simulink model "GS_model"  (R2018b)
settings: Solver=ode5  StartTime=0.0  StopTime=SimuStopTime  FixedStep=T_Simu  RelTol=1e-3
InitFcn:
  | Initial
undefined symbols (not defined in the file or in its folder): Aba10, Aba20, aeroCIP2006_S, aeroCIP2006_X, aeroCIP2006_Y, Agl0, Ass_kS, Ass_n1, Ass_n2, Ass_n3, Ass_n4, Ass_Noise, Ass_R, Ass_Resolution, Ass_TmOrder, AssA_Fix_Abs, AssB_Fix_Abs, AssC_Fix_Abs, AssD_Fix_Abs, AssE_Fix_Aps, AssF_Fix_Aps, C, c_max, c_min, Cd, CenterOfFigNX, CenterOfFigNY, CenterOfFigNZ, CenterOfFigP1, CenterOfFigP2, CenterOfFigPX, CenterOfFigPY, CenterOfFigPZ, Cmu, Crou, DEG2RAD, DiscIntNeverNeededParam, Eg_Dir, Eg_F, Eg_PrepareTime, Eg_r_L_L, Fw_Abf, Fw_Hmax, Fw_J, Fw_Spd0, Fw_Tmax, git_hash_BaseLine, git_hash_Project, Gnss_Noise_Pos, Gnss_Noise_Vel, Gnss_PropgationTime, GyroA_Fix_Abg, GyroA_Noise, GyroB_Fix_Abg, GyroB_Noise, GyroC_Fix_Abg, GyroC_Noise, GyroD_Fix_Abg, GyroD_Noise, h ... (+94)
libraries: simulink x308, sharedutil x46, aerolibutil x37, sharedtransform x31, vrlib x14, aerolibgravity2 x2
(part 4 of 20)

== system GS_model/Subsystem2/EquipmentCmd/Fw1/Subsystem7/Subsystem3 ==
  note: 1 -- FW_Spd_422
      | 2 -- FW_Spd_UDP
      | 3 -- FW_Spd_FC
      |
      | 4 -- FW_T_422
      | 5 -- FW_T_UDP
      | 6 -- FW_T_FC
      |
      | 7 -- FW_Mode_422
      | 8 -- FW_Mode_UDP
      | 9 -- FW_Mode_FC
      |
      | 10--FW_DataSource
  note: FW_DataSource
      | AA-真采集（默认）  1-422(DB9);
      |                                  0-反测（默认
      | 55 -伪采集                UDP
  FWNum : Inport
  FW_Cmd : Inport  Port=2
  TC_Fw : Inport  Port=3
  Compare To Constant : simulink/Logic and Bit Operations/Compare To Constant  relop===  const=0  OutDataTypeStr=boolean
  Demux : Demux  Outputs=[9;1]
  Demux2 : Demux  Outputs=[1;2]
  FWDataSourceChoice : Subsystem
      mask Display: disp('FWDataSourceChoice')
  Logical Operator : Logic  Operator=OR  AllPortsSameDT=off  OutDataTypeStr=boolean
  Mux : Mux  Inputs=3
  Mux1 : Mux  Inputs=2
  Relational Operator1 : RelationalOperator  Operator===  OutDataTypeStr=boolean  RndMeth=Simplest
  Selector : Selector  InputPortWidth=3  IndexOptions=Index vector (dialog)  Indices=[2 3 1]  OutputSizes=1
  Selector2 : Selector  InputPortWidth=23  IndexOptions=Index vector (dialog)  Indices=[1 2]  OutputSizes=1
  Triggered Subsystem1 : Subsystem  TreatAsAtomicUnit=on
      mask Display: disp('FWChoice')
  Cmd_Mode/Spd/T : Outport
  wires:
  Mux/1 -> Cmd_Mode/Spd/T/1
  FWDataSourceChoice/1(Cmd_Mode) -> Mux/1
  Demux/1 -> FWDataSourceChoice/2(FW_Cmd)
  Demux/2 -> Mux1/1
  FW_Cmd/1 -> Demux/1
  TC_Fw/1 -> Selector2/1
  Selector2/1 -> Mux1/2
  FWDataSourceChoice/3(Cmd_T) -> Mux/3
  FWDataSourceChoice/2(Cmd_Spd) -> Mux/2
  Compare To Constant/1 -> Logical Operator/2
  Triggered Subsystem1/1(Out1) -> FWDataSourceChoice/1(FW_Data_Source)
  Mux1/1 -> Selector/1
  Demux2/2 -> Triggered Subsystem1/1(In1)
  Selector/1 -> Demux2/1
  Relational Operator1/1 -> Logical Operator/1
  Logical Operator/1 -> Triggered Subsystem1/Enable
  Demux2/1 -> Compare To Constant/1, Relational Operator1/2
  FWNum/1 -> Relational Operator1/1

== system GS_model/Subsystem2/EquipmentCmd/Fw1/Subsystem7/Subsystem4 ==
  note: FW_DataSource
      | AA-真采集（默认）  1-422(DB9);
      |                                  0-反测（默认
      | 55 -伪采集                UDP
  note: 1 -- FW_Spd_422
      | 2 -- FW_Spd_UDP
      | 3 -- FW_Spd_FC
      |
      | 4 -- FW_T_422
      | 5 -- FW_T_UDP
      | 6 -- FW_T_FC
      |
      | 7 -- FW_Mode_422
      | 8 -- FW_Mode_UDP
      | 9 -- FW_Mode_FC
      |
      | 10--FW_DataSource
  FWNum : Inport
  FW_Cmd : Inport  Port=2
  TC_Fw : Inport  Port=3
  Compare To Constant : simulink/Logic and Bit Operations/Compare To Constant  relop===  const=0  OutDataTypeStr=boolean
  Demux : Demux  Outputs=[9;1]
  Demux2 : Demux  Outputs=[1;2]
  FWDataSourceChoice : Subsystem
      mask Display: disp('FWDataSourceChoice')
  Logical Operator : Logic  Operator=OR  AllPortsSameDT=off  OutDataTypeStr=boolean
  Mux : Mux  Inputs=3
  Mux1 : Mux  Inputs=2
  Relational Operator1 : RelationalOperator  Operator===  OutDataTypeStr=boolean  RndMeth=Simplest
  Selector : Selector  InputPortWidth=3  IndexOptions=Index vector (dialog)  Indices=[2 3 1]  OutputSizes=1
  Selector2 : Selector  InputPortWidth=23  IndexOptions=Index vector (dialog)  Indices=[1 2]  OutputSizes=1
  Triggered Subsystem1 : Subsystem  TreatAsAtomicUnit=on
      mask Display: disp('FWChoice')
  Cmd_Mode/Spd/T : Outport
  wires:
  FWNum/1 -> Relational Operator1/1
  Demux2/1 -> Relational Operator1/2, Compare To Constant/1
  Logical Operator/1 -> Triggered Subsystem1/Enable
  Relational Operator1/1 -> Logical Operator/1
  Selector/1 -> Demux2/1
  Demux2/2 -> Triggered Subsystem1/1(In1)
  Mux1/1 -> Selector/1
  Triggered Subsystem1/1(Out1) -> FWDataSourceChoice/1(FW_Data_Source)
  Compare To Constant/1 -> Logical Operator/2
  FWDataSourceChoice/2(Cmd_Spd) -> Mux/2
  FWDataSourceChoice/3(Cmd_T) -> Mux/3
  Selector2/1 -> Mux1/2
  TC_Fw/1 -> Selector2/1
  FW_Cmd/1 -> Demux/1
  Demux/2 -> Mux1/1
  Demux/1 -> FWDataSourceChoice/2(FW_Cmd)
  FWDataSourceChoice/1(Cmd_Mode) -> Mux/1
  Mux/1 -> Cmd_Mode/Spd/T/1

== system GS_model/Subsystem2/EquipmentCmd/Fw1/Subsystem7/Subsystem5 ==
  note: 1 -- FW_Spd_422
      | 2 -- FW_Spd_UDP
      | 3 -- FW_Spd_FC
      |
      | 4 -- FW_T_422
      | 5 -- FW_T_UDP
      | 6 -- FW_T_FC
      |
      | 7 -- FW_Mode_422
      | 8 -- FW_Mode_UDP
      | 9 -- FW_Mode_FC
      |
      | 10--FW_DataSource
  note: FW_DataSource
      | AA-真采集（默认）  1-422(DB9);
      |                                  0-反测（默认
      | 55 -伪采集                UDP
  FWNum : Inport
  FW_Cmd : Inport  Port=2
  TC_Fw : Inport  Port=3
  Compare To Constant : simulink/Logic and Bit Operations/Compare To Constant  relop===  const=0  OutDataTypeStr=boolean
  Demux : Demux  Outputs=[9;1]
  Demux2 : Demux  Outputs=[1;2]
  FWDataSourceChoice : Subsystem
      mask Display: disp('FWDataSourceChoice')
  Logical Operator : Logic  Operator=OR  AllPortsSameDT=off  OutDataTypeStr=boolean
  Mux : Mux  Inputs=3
  Mux1 : Mux  Inputs=2
  Relational Operator1 : RelationalOperator  Operator===  OutDataTypeStr=boolean  RndMeth=Simplest
  Selector : Selector  InputPortWidth=3  IndexOptions=Index vector (dialog)  Indices=[2 3 1]  OutputSizes=1
  Selector2 : Selector  InputPortWidth=23  IndexOptions=Index vector (dialog)  Indices=[1 2]  OutputSizes=1
  Triggered Subsystem1 : Subsystem  TreatAsAtomicUnit=on
      mask Display: disp('FWChoice')
  Cmd_Mode/Spd/T : Outport
  wires:
  Mux/1 -> Cmd_Mode/Spd/T/1
  FWDataSourceChoice/1(Cmd_Mode) -> Mux/1
  Demux/1 -> FWDataSourceChoice/2(FW_Cmd)
  Demux/2 -> Mux1/1
  FW_Cmd/1 -> Demux/1
  TC_Fw/1 -> Selector2/1
  Selector2/1 -> Mux1/2
  FWDataSourceChoice/3(Cmd_T) -> Mux/3
  FWDataSourceChoice/2(Cmd_Spd) -> Mux/2
  Compare To Constant/1 -> Logical Operator/2
  Triggered Subsystem1/1(Out1) -> FWDataSourceChoice/1(FW_Data_Source)
  Mux1/1 -> Selector/1
  Demux2/2 -> Triggered Subsystem1/1(In1)
  Selector/1 -> Demux2/1
  Relational Operator1/1 -> Logical Operator/1
  Logical Operator/1 -> Triggered Subsystem1/Enable
  Demux2/1 -> Compare To Constant/1, Relational Operator1/2
  FWNum/1 -> Relational Operator1/1

== system GS_model/Subsystem2/EquipmentCmd/Fw1/Subsystem7/Subsystem6 ==
  note: FW_DataSource
      | AA-真采集（默认）  1-422(DB9);
      |                                  0-反测（默认
      | 55 -伪采集                UDP
  note: 1 -- FW_Spd_422
      | 2 -- FW_Spd_UDP
      | 3 -- FW_Spd_FC
      |
      | 4 -- FW_T_422
      | 5 -- FW_T_UDP
      | 6 -- FW_T_FC
      |
      | 7 -- FW_Mode_422
      | 8 -- FW_Mode_UDP
      | 9 -- FW_Mode_FC
      |
      | 10--FW_DataSource
  FWNum : Inport
  FW_Cmd : Inport  Port=2
  TC_Fw : Inport  Port=3
  Compare To Constant : simulink/Logic and Bit Operations/Compare To Constant  relop===  const=0  OutDataTypeStr=boolean
  Demux : Demux  Outputs=[9;1]
  Demux2 : Demux  Outputs=[1;2]
  FWDataSourceChoice : Subsystem
      mask Display: disp('FWDataSourceChoice')
  Logical Operator : Logic  Operator=OR  AllPortsSameDT=off  OutDataTypeStr=boolean
  Mux : Mux  Inputs=3
  Mux1 : Mux  Inputs=2
  Relational Operator1 : RelationalOperator  Operator===  OutDataTypeStr=boolean  RndMeth=Simplest
  Selector : Selector  InputPortWidth=3  IndexOptions=Index vector (dialog)  Indices=[2 3 1]  OutputSizes=1
  Selector2 : Selector  InputPortWidth=23  IndexOptions=Index vector (dialog)  Indices=[1 2]  OutputSizes=1
  Triggered Subsystem1 : Subsystem  TreatAsAtomicUnit=on
      mask Display: disp('FWChoice')
  Cmd_Mode/Spd/T : Outport
  wires:
  FWNum/1 -> Relational Operator1/1
  Demux2/1 -> Relational Operator1/2, Compare To Constant/1
  Logical Operator/1 -> Triggered Subsystem1/Enable
  Relational Operator1/1 -> Logical Operator/1
  Selector/1 -> Demux2/1
  Demux2/2 -> Triggered Subsystem1/1(In1)
  Mux1/1 -> Selector/1
  Triggered Subsystem1/1(Out1) -> FWDataSourceChoice/1(FW_Data_Source)
  Compare To Constant/1 -> Logical Operator/2
  FWDataSourceChoice/2(Cmd_Spd) -> Mux/2
  FWDataSourceChoice/3(Cmd_T) -> Mux/3
  Selector2/1 -> Mux1/2
  TC_Fw/1 -> Selector2/1
  FW_Cmd/1 -> Demux/1
  Demux/2 -> Mux1/1
  Demux/1 -> FWDataSourceChoice/2(FW_Cmd)
  FWDataSourceChoice/1(Cmd_Mode) -> Mux/1
  Mux/1 -> Cmd_Mode/Spd/T/1

== system GS_model/Subsystem2/Subsystem/Actuator/Engine/Subsystem ==
  note: F_Choice/Switch/Value
  note: Dir_Choice/Switch/X/Y/Z
  note: FirePause_Choice/Switch/Value
  Tc_F_Engine : Inport
  Cmd_Engine : Inport  Port=2
  Cent : Inport  Port=3
  Eg_F : Inport  Port=4
  Eg_PrepareTime : Inport  Port=5
  Eg_r_L_L : Inport  Port=6
  Eg_Dir : Inport  Port=7
  EgNum : Inport  Port=8
  Demux1 : Demux  Outputs=[5;3;3]
  Engine : Subsystem
      mask Display: disp('EngineModel')
  Fcn : Fcn  Expr=3*u(1)-2
  Fcn1 : Fcn  Expr=3*u(1)-2
  Fcn2 : Fcn  Expr=2*u(1)-1
  Fcn3 : Fcn  Expr=2*u(1)
  Selector1 : Selector  InputPortWidth=size(Eg_F,1)  IndexOptions=Starting index (port)  Indices=[1 3]  OutputSizes=1
  Selector14 : Selector  InputPortWidth=size(Eg_F,1)*2  IndexOptions=Starting index (port)  Indices=[1 3]  OutputSizes=1
  Selector2 : Selector  InputPortWidth=size(Eg_F,1)  IndexOptions=Starting index (port)  Indices=[1 3]  OutputSizes=1
  Selector3 : Selector  InputPortWidth=size(Eg_F,1)*3  IndexOptions=Starting index (port)  Indices=[1 3]  OutputSizes=3
  Selector4 : Selector  InputPortWidth=size(Eg_F,1)*3  IndexOptions=Starting index (port)  Indices=[1 3]  OutputSizes=3
  Selector5 : Selector  InputPortWidth=size(Eg_F,1)*2  IndexOptions=Starting index (port)  Indices=[1 3]  OutputSizes=1
  Subsystem : Subsystem
  Subsystem1 : Subsystem
  Subsystem2 : Subsystem
  T : Outport
  F : Outport  Port=2
  wires:
  Engine/2(F_EP) -> F/1
  Engine/1(T_Engine) -> T/1
  EgNum/1 -> Fcn2/1, Fcn3/1, Selector1/2, Subsystem2/2(Num), Subsystem1/3(Num), Subsystem/3(Num), Selector2/2, Fcn1/1, Fcn/1
  Cent/1 -> Engine/5(Cent)
  Eg_PrepareTime/1 -> Selector1/1
  Tc_F_Engine/1 -> Demux1/1
  Demux1/2 -> Subsystem1/2(Eg_F_Set)
  Eg_r_L_L/1 -> Selector3/1
  Fcn/1 -> Selector3/2
  Selector1/1 -> Engine/3(Eg_PrepareTime)
  Selector3/1 -> Engine/4(Eg_r_L_L)
  Fcn1/1 -> Selector4/2
  Eg_Dir/1 -> Selector4/1
  Selector4/1 -> Subsystem/1(Eg_Dir0)
  Demux1/1 -> Subsystem/2(Eg_Dir_Set)
  Selector2/1 -> Subsystem1/1(Eg_F0)
  Eg_F/1 -> Selector2/1
  Subsystem/1(Eg_Dir) -> Engine/6(Eg_Dir)
  Subsystem1/1(Eg_F) -> Engine/7(Eg_F)
  Fcn2/1 -> Selector5/2
  Fcn3/1 -> Selector14/2
  Cmd_Engine/1 -> Selector14/1, Selector5/1
  Selector5/1 -> Engine/1(FireSwitch)
  Selector14/1 -> Engine/2(FireTime)
  Demux1/3 -> Subsystem2/1(Eg_F_Set)
  Subsystem2/1(Eg_FirePause) -> Engine/8(Eg_Fire_Pause)

== system GS_model/Subsystem2/Subsystem/Actuator/Engine/Subsystem1 ==
  note: FirePause_Choice/Switch/Value
  note: Dir_Choice/Switch/X/Y/Z
  note: F_Choice/Switch/Value
  Tc_F_Engine : Inport
  Cmd_Engine : Inport  Port=2
  Cent : Inport  Port=3
  Eg_F : Inport  Port=4
  Eg_PrepareTime : Inport  Port=5
  Eg_r_L_L : Inport  Port=6
  Eg_Dir : Inport  Port=7
  EgNum : Inport  Port=8
  Demux1 : Demux  Outputs=[5;3;3]
  Engine : Subsystem
      mask Display: disp('EngineModel')
  Fcn : Fcn  Expr=3*u(1)-2
  Fcn1 : Fcn  Expr=3*u(1)-2
  Fcn2 : Fcn  Expr=2*u(1)-1
  Fcn3 : Fcn  Expr=2*u(1)
  Selector1 : Selector  InputPortWidth=size(Eg_F,1)  IndexOptions=Starting index (port)  Indices=[1 3]  OutputSizes=1
  Selector14 : Selector  InputPortWidth=size(Eg_F,1)*2  IndexOptions=Starting index (port)  Indices=[1 3]  OutputSizes=1
  Selector2 : Selector  InputPortWidth=size(Eg_F,1)  IndexOptions=Starting index (port)  Indices=[1 3]  OutputSizes=1
  Selector3 : Selector  InputPortWidth=size(Eg_F,1)*3  IndexOptions=Starting index (port)  Indices=[1 3]  OutputSizes=3
  Selector4 : Selector  InputPortWidth=size(Eg_F,1)*3  IndexOptions=Starting index (port)  Indices=[1 3]  OutputSizes=3
  Selector5 : Selector  InputPortWidth=size(Eg_F,1)*2  IndexOptions=Starting index (port)  Indices=[1 3]  OutputSizes=1
  Subsystem : Subsystem
  Subsystem1 : Subsystem
  Subsystem2 : Subsystem
  T : Outport
  F : Outport  Port=2
  wires:
  Subsystem2/1(Eg_FirePause) -> Engine/8(Eg_Fire_Pause)
  Demux1/3 -> Subsystem2/1(Eg_F_Set)
  Selector14/1 -> Engine/2(FireTime)
  Selector5/1 -> Engine/1(FireSwitch)
  Cmd_Engine/1 -> Selector5/1, Selector14/1
  Fcn3/1 -> Selector14/2
  Fcn2/1 -> Selector5/2
  Subsystem1/1(Eg_F) -> Engine/7(Eg_F)
  Subsystem/1(Eg_Dir) -> Engine/6(Eg_Dir)
  Eg_F/1 -> Selector2/1
  Selector2/1 -> Subsystem1/1(Eg_F0)
  Demux1/1 -> Subsystem/2(Eg_Dir_Set)
  Selector4/1 -> Subsystem/1(Eg_Dir0)
  Eg_Dir/1 -> Selector4/1
  Fcn1/1 -> Selector4/2
  Selector3/1 -> Engine/4(Eg_r_L_L)
  Selector1/1 -> Engine/3(Eg_PrepareTime)
  Fcn/1 -> Selector3/2
  Eg_r_L_L/1 -> Selector3/1
  Demux1/2 -> Subsystem1/2(Eg_F_Set)
  Tc_F_Engine/1 -> Demux1/1
  Eg_PrepareTime/1 -> Selector1/1
  Cent/1 -> Engine/5(Cent)
  EgNum/1 -> Fcn/1, Fcn1/1, Selector2/2, Subsystem/3(Num), Subsystem1/3(Num), Subsystem2/2(Num), Selector1/2, Fcn3/1, Fcn2/1
  Engine/1(T_Engine) -> T/1
  Engine/2(F_EP) -> F/1

== system GS_model/Subsystem2/Subsystem/Actuator/FlyWheel/FwAModel1 ==
  note: TC_FW_DelaySet[1*1]
  note: 1 -- TM_FW_Mode
      | 2 -- TM_FW_Spd
      | 3 -- TM_FW_T
      |
      | 4 -- Cmd_FW_Mode
      | 5 -- Cmd_FW_Spd
      | 6 -- Cmd_FW_T
      |
      | 7 -- Dyn_FW_T
      | 8 -- Dyn_FW_Spd
  note: TC_FW_TSet[3*1]
  note: TC_FW_SpdSet[3*1]
  note: TC_FW_ModeSet[3*1]
  note: TC_FWErr_Spd_Op[2*1]
  note: TC_FWErr_T_Op[2*1]
  note: Tc_FW_FricCoffSet[1*1]
  FW_Cmd : Inport
  TC_FW : Inport  Port=2
  FwSpd/T : Inport  Port=3
  FWNum : Inport  Port=4
  Demux : Demux  Outputs=2
  Demux1 : Demux  Outputs=[1;3;3;3;2;2;1]
  FWDataSourceChoice : Subsystem
      mask Display: disp('FWDataSourceChoice')
  FWMath&ErrModel : Subsystem
      mask Display: disp('FWMath&ErrModel')
  Mux : Mux
  Terminator : Terminator
  TM_FW : Outport
  Cmd_Mode/Spd/T : Outport  Port=2
  wires:
  FwSpd/T/1 -> Demux/1
  Demux/2 -> FWMath&ErrModel/8(FwT)
  Demux/1 -> FWMath&ErrModel/7(FwSpd)
  Demux1/7 -> Terminator/1
  FWDataSourceChoice/1(Cmd_Mode/Spd/T) -> Mux/2, Cmd_Mode/Spd/T/1
  Demux1/1 -> FWDataSourceChoice/2(TC_FW_DelaySet)
  FW_Cmd/1 -> FWDataSourceChoice/1(FW_Cmd)
  TC_FW/1 -> Demux1/1
  FWDataSourceChoice/2(Cmd_Mode) -> FWMath&ErrModel/1(Cmd_Mode)
  FWNum/1 -> FWMath&ErrModel/9(FWNum)
  FWMath&ErrModel/1(TM_FW) -> Mux/1
  Demux1/6 -> FWMath&ErrModel/6(TC_FWErr_T_Op)
  Demux1/5 -> FWMath&ErrModel/5(TC_FWErr_Spd_Op)
  Demux1/4 -> FWMath&ErrModel/4(TC_FW_ModeSet)
  Demux1/3 -> FWMath&ErrModel/3(TC_FW_SpdSet)
  Demux1/2 -> FWMath&ErrModel/2(TC_FW_TSet)
  FWMath&ErrModel/2(Dyn_FW_T) -> Mux/3
  Mux/1 -> TM_FW/1
  FWMath&ErrModel/3(Dyn_FW_Spd) -> Mux/4

== system GS_model/Subsystem2/Subsystem/Actuator/FlyWheel/FwAModel2 ==
  note: Tc_FW_FricCoffSet[1*1]
  note: TC_FWErr_T_Op[2*1]
  note: TC_FWErr_Spd_Op[2*1]
  note: TC_FW_ModeSet[3*1]
  note: TC_FW_SpdSet[3*1]
  note: TC_FW_TSet[3*1]
  note: 1 -- TM_FW_Mode
      | 2 -- TM_FW_Spd
      | 3 -- TM_FW_T
      |
      | 4 -- Cmd_FW_Mode
      | 5 -- Cmd_FW_Spd
      | 6 -- Cmd_FW_T
      |
      | 7 -- Dyn_FW_T
      | 8 -- Dyn_FW_Spd
  note: TC_FW_DelaySet[1*1]
  FW_Cmd : Inport
  TC_FW : Inport  Port=2
  FwSpd/T : Inport  Port=3
  FWNum : Inport  Port=4
  Demux : Demux  Outputs=2
  Demux1 : Demux  Outputs=[1;3;3;3;2;2;1]
  FWDataSourceChoice : Subsystem
      mask Display: disp('FWDataSourceChoice')
  FWMath&ErrModel : Subsystem
      mask Display: disp('FWMath&ErrModel')
  Mux : Mux
  Terminator : Terminator
  TM_FW : Outport
  Cmd_Mode/Spd/T : Outport  Port=2
  wires:
  FWMath&ErrModel/3(Dyn_FW_Spd) -> Mux/4
  Mux/1 -> TM_FW/1
  FWMath&ErrModel/2(Dyn_FW_T) -> Mux/3
  Demux1/2 -> FWMath&ErrModel/2(TC_FW_TSet)
  Demux1/3 -> FWMath&ErrModel/3(TC_FW_SpdSet)
  Demux1/4 -> FWMath&ErrModel/4(TC_FW_ModeSet)
  Demux1/5 -> FWMath&ErrModel/5(TC_FWErr_Spd_Op)
  Demux1/6 -> FWMath&ErrModel/6(TC_FWErr_T_Op)
  FWMath&ErrModel/1(TM_FW) -> Mux/1
  FWNum/1 -> FWMath&ErrModel/9(FWNum)
  FWDataSourceChoice/2(Cmd_Mode) -> FWMath&ErrModel/1(Cmd_Mode)
  TC_FW/1 -> Demux1/1
  FW_Cmd/1 -> FWDataSourceChoice/1(FW_Cmd)
  Demux1/1 -> FWDataSourceChoice/2(TC_FW_DelaySet)
  FWDataSourceChoice/1(Cmd_Mode/Spd/T) -> Cmd_Mode/Spd/T/1, Mux/2
  Demux1/7 -> Terminator/1
  Demux/1 -> FWMath&ErrModel/7(FwSpd)
  Demux/2 -> FWMath&ErrModel/8(FwT)
  FwSpd/T/1 -> Demux/1

== system GS_model/Subsystem2/Subsystem/Actuator/FlyWheel/FwAModel3 ==
  note: TC_FW_DelaySet[1*1]
  note: 1 -- TM_FW_Mode
      | 2 -- TM_FW_Spd
      | 3 -- TM_FW_T
      |
      | 4 -- Cmd_FW_Mode
      | 5 -- Cmd_FW_Spd
      | 6 -- Cmd_FW_T
      |
      | 7 -- Dyn_FW_T
      | 8 -- Dyn_FW_Spd
  note: TC_FW_TSet[3*1]
  note: TC_FW_SpdSet[3*1]
  note: TC_FW_ModeSet[3*1]
  note: TC_FWErr_Spd_Op[2*1]
  note: TC_FWErr_T_Op[2*1]
  note: Tc_FW_FricCoffSet[1*1]
  FW_Cmd : Inport
  TC_FW : Inport  Port=2
  FwSpd/T : Inport  Port=3
  FWNum : Inport  Port=4
  Demux : Demux  Outputs=2
  Demux1 : Demux  Outputs=[1;3;3;3;2;2;1]
  FWDataSourceChoice : Subsystem
      mask Display: disp('FWDataSourceChoice')
  FWMath&ErrModel : Subsystem
      mask Display: disp('FWMath&ErrModel')
  Mux : Mux
  Terminator : Terminator
  TM_FW : Outport
  Cmd_Mode/Spd/T : Outport  Port=2
  wires:
  FwSpd/T/1 -> Demux/1
  Demux/2 -> FWMath&ErrModel/8(FwT)
  Demux/1 -> FWMath&ErrModel/7(FwSpd)
  Demux1/7 -> Terminator/1
  FWDataSourceChoice/1(Cmd_Mode/Spd/T) -> Mux/2, Cmd_Mode/Spd/T/1
  Demux1/1 -> FWDataSourceChoice/2(TC_FW_DelaySet)
  FW_Cmd/1 -> FWDataSourceChoice/1(FW_Cmd)
  TC_FW/1 -> Demux1/1
  FWDataSourceChoice/2(Cmd_Mode) -> FWMath&ErrModel/1(Cmd_Mode)
  FWNum/1 -> FWMath&ErrModel/9(FWNum)
  FWMath&ErrModel/1(TM_FW) -> Mux/1
  Demux1/6 -> FWMath&ErrModel/6(TC_FWErr_T_Op)
  Demux1/5 -> FWMath&ErrModel/5(TC_FWErr_Spd_Op)
  Demux1/4 -> FWMath&ErrModel/4(TC_FW_ModeSet)
  Demux1/3 -> FWMath&ErrModel/3(TC_FW_SpdSet)
  Demux1/2 -> FWMath&ErrModel/2(TC_FW_TSet)
  FWMath&ErrModel/2(Dyn_FW_T) -> Mux/3
  Mux/1 -> TM_FW/1
  FWMath&ErrModel/3(Dyn_FW_Spd) -> Mux/4

== system GS_model/Subsystem2/Subsystem/Actuator/FlyWheel/FwAModel4 ==
  note: Tc_FW_FricCoffSet[1*1]
  note: TC_FWErr_T_Op[2*1]
  note: TC_FWErr_Spd_Op[2*1]
  note: TC_FW_ModeSet[3*1]
  note: TC_FW_SpdSet[3*1]
  note: TC_FW_TSet[3*1]
  note: 1 -- TM_FW_Mode
      | 2 -- TM_FW_Spd
      | 3 -- TM_FW_T
      |
      | 4 -- Cmd_FW_Mode
      | 5 -- Cmd_FW_Spd
      | 6 -- Cmd_FW_T
      |
      | 7 -- Dyn_FW_T
      | 8 -- Dyn_FW_Spd
  note: TC_FW_DelaySet[1*1]
  FW_Cmd : Inport
  TC_FW : Inport  Port=2
  FwSpd/T : Inport  Port=3
  FWNum : Inport  Port=4
  Demux : Demux  Outputs=2
  Demux1 : Demux  Outputs=[1;3;3;3;2;2;1]
  FWDataSourceChoice : Subsystem
      mask Display: disp('FWDataSourceChoice')
  FWMath&ErrModel : Subsystem
      mask Display: disp('FWMath&ErrModel')
  Mux : Mux
  Terminator : Terminator
  TM_FW : Outport
  Cmd_Mode/Spd/T : Outport  Port=2
  wires:
  FWMath&ErrModel/3(Dyn_FW_Spd) -> Mux/4
  Mux/1 -> TM_FW/1
  FWMath&ErrModel/2(Dyn_FW_T) -> Mux/3
  Demux1/2 -> FWMath&ErrModel/2(TC_FW_TSet)
  Demux1/3 -> FWMath&ErrModel/3(TC_FW_SpdSet)
  Demux1/4 -> FWMath&ErrModel/4(TC_FW_ModeSet)
  Demux1/5 -> FWMath&ErrModel/5(TC_FWErr_Spd_Op)
  Demux1/6 -> FWMath&ErrModel/6(TC_FWErr_T_Op)
  FWMath&ErrModel/1(TM_FW) -> Mux/1
  FWNum/1 -> FWMath&ErrModel/9(FWNum)
  FWDataSourceChoice/2(Cmd_Mode) -> FWMath&ErrModel/1(Cmd_Mode)
  TC_FW/1 -> Demux1/1
  FW_Cmd/1 -> FWDataSourceChoice/1(FW_Cmd)
  Demux1/1 -> FWDataSourceChoice/2(TC_FW_DelaySet)
  FWDataSourceChoice/1(Cmd_Mode/Spd/T) -> Cmd_Mode/Spd/T/1, Mux/2
  Demux1/7 -> Terminator/1
  Demux/1 -> FWMath&ErrModel/7(FwSpd)
  Demux/2 -> FWMath&ErrModel/8(FwT)
  FwSpd/T/1 -> Demux/1

== system GS_model/Subsystem2/Subsystem/Actuator/FlyWheel/FwAModel5 ==
  note: TC_FW_DelaySet[1*1]
  note: 1 -- TM_FW_Mode
      | 2 -- TM_FW_Spd
      | 3 -- TM_FW_T
      |
      | 4 -- Cmd_FW_Mode
      | 5 -- Cmd_FW_Spd
      | 6 -- Cmd_FW_T
      |
      | 7 -- Dyn_FW_T
      | 8 -- Dyn_FW_Spd
  note: TC_FW_TSet[3*1]
  note: TC_FW_SpdSet[3*1]
  note: TC_FW_ModeSet[3*1]
  note: TC_FWErr_Spd_Op[2*1]
  note: TC_FWErr_T_Op[2*1]
  note: Tc_FW_FricCoffSet[1*1]
  FW_Cmd : Inport
  TC_FW : Inport  Port=2
  FwSpd/T : Inport  Port=3
  FWNum : Inport  Port=4
  Demux : Demux  Outputs=2
  Demux1 : Demux  Outputs=[1;3;3;3;2;2;1]
  FWDataSourceChoice : Subsystem
      mask Display: disp('FWDataSourceChoice')
  FWMath&ErrModel : Subsystem
      mask Display: disp('FWMath&ErrModel')
  Mux : Mux
  Terminator : Terminator
  TM_FW : Outport
  Cmd_Mode/Spd/T : Outport  Port=2
  wires:
  FwSpd/T/1 -> Demux/1
  Demux/2 -> FWMath&ErrModel/8(FwT)
  Demux/1 -> FWMath&ErrModel/7(FwSpd)
  Demux1/7 -> Terminator/1
  FWDataSourceChoice/1(Cmd_Mode/Spd/T) -> Mux/2, Cmd_Mode/Spd/T/1
  Demux1/1 -> FWDataSourceChoice/2(TC_FW_DelaySet)
  FW_Cmd/1 -> FWDataSourceChoice/1(FW_Cmd)
  TC_FW/1 -> Demux1/1
  FWDataSourceChoice/2(Cmd_Mode) -> FWMath&ErrModel/1(Cmd_Mode)
  FWNum/1 -> FWMath&ErrModel/9(FWNum)
  FWMath&ErrModel/1(TM_FW) -> Mux/1
  Demux1/6 -> FWMath&ErrModel/6(TC_FWErr_T_Op)
  Demux1/5 -> FWMath&ErrModel/5(TC_FWErr_Spd_Op)
  Demux1/4 -> FWMath&ErrModel/4(TC_FW_ModeSet)
  Demux1/3 -> FWMath&ErrModel/3(TC_FW_SpdSet)
  Demux1/2 -> FWMath&ErrModel/2(TC_FW_TSet)
  FWMath&ErrModel/2(Dyn_FW_T) -> Mux/3
  Mux/1 -> TM_FW/1
  FWMath&ErrModel/3(Dyn_FW_Spd) -> Mux/4

== system GS_model/Subsystem2/Subsystem/Actuator/FlyWheel/FwAModel6 ==
  note: Tc_FW_FricCoffSet[1*1]
  note: TC_FWErr_T_Op[2*1]
  note: TC_FWErr_Spd_Op[2*1]
  note: TC_FW_ModeSet[3*1]
  note: TC_FW_SpdSet[3*1]
  note: TC_FW_TSet[3*1]
  note: 1 -- TM_FW_Mode
      | 2 -- TM_FW_Spd
      | 3 -- TM_FW_T
      |
      | 4 -- Cmd_FW_Mode
      | 5 -- Cmd_FW_Spd
      | 6 -- Cmd_FW_T
      |
      | 7 -- Dyn_FW_T
      | 8 -- Dyn_FW_Spd
  note: TC_FW_DelaySet[1*1]
  FW_Cmd : Inport
  TC_FW : Inport  Port=2
  FwSpd/T : Inport  Port=3
  FWNum : Inport  Port=4
  Demux : Demux  Outputs=2
  Demux1 : Demux  Outputs=[1;3;3;3;2;2;1]
  FWDataSourceChoice : Subsystem
      mask Display: disp('FWDataSourceChoice')
  FWMath&ErrModel : Subsystem
      mask Display: disp('FWMath&ErrModel')
  Mux : Mux
  Terminator : Terminator
  TM_FW : Outport
  Cmd_Mode/Spd/T : Outport  Port=2
  wires:
  FWMath&ErrModel/3(Dyn_FW_Spd) -> Mux/4
  Mux/1 -> TM_FW/1
  FWMath&ErrModel/2(Dyn_FW_T) -> Mux/3
  Demux1/2 -> FWMath&ErrModel/2(TC_FW_TSet)
  Demux1/3 -> FWMath&ErrModel/3(TC_FW_SpdSet)
  Demux1/4 -> FWMath&ErrModel/4(TC_FW_ModeSet)
  Demux1/5 -> FWMath&ErrModel/5(TC_FWErr_Spd_Op)
  Demux1/6 -> FWMath&ErrModel/6(TC_FWErr_T_Op)
  FWMath&ErrModel/1(TM_FW) -> Mux/1
  FWNum/1 -> FWMath&ErrModel/9(FWNum)
  FWDataSourceChoice/2(Cmd_Mode) -> FWMath&ErrModel/1(Cmd_Mode)
  TC_FW/1 -> Demux1/1
  FW_Cmd/1 -> FWDataSourceChoice/1(FW_Cmd)
  Demux1/1 -> FWDataSourceChoice/2(TC_FW_DelaySet)
  FWDataSourceChoice/1(Cmd_Mode/Spd/T) -> Cmd_Mode/Spd/T/1, Mux/2
  Demux1/7 -> Terminator/1
  Demux/1 -> FWMath&ErrModel/7(FwSpd)
  Demux/2 -> FWMath&ErrModel/8(FwT)
  FwSpd/T/1 -> Demux/1

== system GS_model/Subsystem2/Subsystem/Actuator/FlyWheel/FwAModel7 ==
  FwSpd0 : Inport
  Tc_FW_FricCoffSet : Inport  Port=2
  Cmd_FwABCDEF : Inport  Port=3
  AttReset : Inport  Port=4
  FwMathModel : Subsystem
      mask Display: disp('FwMathModel')
  Selector : Selector  InputPortWidth=18  IndexOptions=Index vector (dialog)  Indices=[1:3:18]  OutputSizes=1
  Selector1 : Selector  InputPortWidth=18  IndexOptions=Index vector (dialog)  Indices=[2:3:18]  OutputSizes=1
  Selector2 : Selector  InputPortWidth=18  IndexOptions=Index vector (dialog)  Indices=[3:3:18]  OutputSizes=1
  Selector6 : Selector  InputPortWidth=23  IndexOptions=Index vector (dialog)  Indices=[18:23]  OutputSizes=1
  Fw_Spd_out : Outport
  Fw_T_out : Outport  Port=2
  wires:
  Cmd_FwABCDEF/1 -> Selector2/1, Selector1/1, Selector/1
  Selector/1 -> FwMathModel/1(Cmd_Mode)
  Selector1/1 -> FwMathModel/2(Cmd_Spd)
  Selector2/1 -> FwMathModel/3(Cmd_T)
  AttReset/1 -> FwMathModel/4(Reset)
  FwSpd0/1 -> Selector6/1
  Tc_FW_FricCoffSet/1 -> FwMathModel/6(Tc_Fw_FricCoff)
  FwMathModel/1(Fw_Spd_out) -> Fw_Spd_out/1
  FwMathModel/2(Fw_T_out) -> Fw_T_out/1
  Selector6/1 -> FwMathModel/5(FwH0)

== system GS_model/Subsystem2/Subsystem/Actuator/Magnetorquer/Mt_MathModel ==
  note: Val1 Dir1 Val2 Dir2 ....
  note: TC_MtCoffSet[6*1]
  note: TC_MtGNDSet[3*1]
  Cmd_Mt_Pro : Inport
  Tc_Mt : Inport  Port=2
  Constant1 : Constant  Value=2
  Constant2 : Constant
  Constant3 : Constant  Value=3
  Constant4 : Constant  Value=5
  Constant5 : Constant  Value=4
  Constant6 : Constant  Value=6
  Demux : Demux  Outputs=[6;3]
  Demux2 : Demux  Outputs=[2;2;2;2;2;2]
  MtA1 : Subsystem
  MtA2 : Subsystem
  MtA3 : Subsystem
  MtA4 : Subsystem
  MtA5 : Subsystem
  MtA6 : Subsystem
  Mux1 : Mux  Inputs=6
  Mux2 : Mux  Inputs=6
  Mux3 : Mux  Inputs=6
  Product11 : Product  SaturateOnIntegerOverflow=on  OutDataTypeStr=Inherit: Same as first input
  M_Mt : Outport
  Cmd_Mt : Outport  Port=2
  Tm_Mt : Outport  Port=3
  wires:
  Product11/1 -> M_Mt/1
  Mux1/1 -> Cmd_Mt/1
  Cmd_Mt_Pro/1 -> Demux2/1
  Mux3/1 -> Product11/2
  Mux2/1 -> Tm_Mt/1
  Constant2/1 -> MtA1/3(Mt_Num)
  Constant1/1 -> MtA2/3(Mt_Num)
  Demux/2 -> MtA2/1(Tc_Mt), MtA3/1(Tc_Mt), MtA4/1(Tc_Mt), MtA6/1(Tc_Mt), MtA5/1(Tc_Mt), MtA1/1(Tc_Mt)
  MtA1/1(Mc_Mt) -> Mux3/1
  Tc_Mt/1 -> Demux/1
  Demux/1 -> Product11/1
  Demux2/2 -> MtA2/2(Cmd)
  Demux2/1 -> MtA1/2(Cmd)
  Demux2/3 -> MtA3/2(Cmd)
  Demux2/4 -> MtA4/2(Cmd)
  Demux2/5 -> MtA5/2(Cmd)
  Demux2/6 -> MtA6/2(Cmd)
  Constant3/1 -> MtA3/3(Mt_Num)
  Constant4/1 -> MtA5/3(Mt_Num)
  Constant6/1 -> MtA6/3(Mt_Num)
  Constant5/1 -> MtA4/3(Mt_Num)
  MtA2/1(Mc_Mt) -> Mux3/2
  MtA3/1(Mc_Mt) -> Mux3/3
  MtA4/1(Mc_Mt) -> Mux3/4
  MtA5/1(Mc_Mt) -> Mux3/5
  MtA6/1(Mc_Mt) -> Mux3/6
  MtA1/2(Tm_Mt) -> Mux2/1
  MtA2/2(Tm_Mt) -> Mux2/2
  MtA3/2(Tm_Mt) -> Mux2/3
  MtA4/2(Tm_Mt) -> Mux2/4
  MtA5/2(Tm_Mt) -> Mux2/5
  MtA6/2(Tm_Mt) -> Mux2/6
  MtA6/3(Cmd_Mt) -> Mux1/6
  MtA1/3(Cmd_Mt) -> Mux1/1
  MtA2/3(Cmd_Mt) -> Mux1/2
  MtA3/3(Cmd_Mt) -> Mux1/3
  MtA4/3(Cmd_Mt) -> Mux1/4
  MtA5/3(Cmd_Mt) -> Mux1/5

== system GS_model/Subsystem2/Subsystem/Actuator/Motor/QV ==
  note: Agl_A/B/C/D
      | W_A/B/C/D
      | a_A/B/C/D
  note: Agl/w/a_A
      | Agl/w/a_B
      | Agl/w/a_C
      | Agl/w/a_D
  TC_Motor_in : Inport
  Cmd_Motor_in : Inport  Port=2
  AttReset : Inport  Port=3
  QVAgl_FC : Inport  Port=4
  UTC_1970 : Inport  Port=5
  Agl2Agl/w/a : Subsystem
  Constant : Constant  Value=QV_XbLw_Value
  Constant5 : Constant  Value=360
  Data_QV : Subsystem
  Fre_QV : Subsystem
  Integrator : Integrator  ExternalReset=level  InitialConditionSource=external  LimitOutput=on  UpperSaturationLimit=max([(QV_A_RotUnitQV.*QV_PosLocationLimit_Real) (QV_A_RotUnitQV.*QV_NegLocationLimit_Real)],[],2)  LowerSaturationLimit=min([(QV_A_RotUnitQV.*QV_PosLocationLimit_Real) (QV_A_RotUnitQV.*QV_NegLocationLimit_Real)],[],2)
  Limit±180deg : Subsystem
  MATLAB Function4 : MATLAB Function  TreatAsAtomicUnit=on
  Mod : Math  Operator=mod  SaturateOnIntegerOverflow=on
  Mux : Mux  Inputs=2
  Mux2 : Mux  Inputs=5
  QV_A_DriveRotUnit : Gain  Gain=QV_A_DriveRotUnit  SaturateOnIntegerOverflow=on  OutDataTypeStr=Inherit: Same as input  ParamDataTypeStr=Inherit: Same as input
  "QV_A_DriveRotunit " : Gain  Gain=QV_A_DriveRotUnit  SaturateOnIntegerOverflow=on  OutDataTypeStr=Inherit: Same as input  ParamDataTypeStr=Inherit: Same as input
  QV_A_RotUnitQV : Gain  Gain=QV_A_RotUnitQV  SaturateOnIntegerOverflow=on  OutDataTypeStr=Inherit: Same as input  ParamDataTypeStr=Inherit: Same as input
  "QV_A_RotUnitQV " : Gain  Gain=QV_A_RotUnitQV  SaturateOnIntegerOverflow=on  OutDataTypeStr=Inherit: Same as input  ParamDataTypeStr=Inherit: Same as input
  Selector : Selector  InputPortWidth=17  IndexOptions=Index vector (dialog)  Indices=[5:9]  OutputSizes=1
  Selector1 : Selector  InputPortWidth=12  IndexOptions=Index vector (dialog)  Indices=[1 5 9 2 6 10 3 7 11 4 8 12]  OutputSizes=1
  Selector2 : Selector  InputPortWidth=17  IndexOptions=Index vector (dialog)  Indices=[10:13]  OutputSizes=1
  Selector3 : Selector  InputPortWidth=17  IndexOptions=Index vector (dialog)  Indices=[1:9]  OutputSizes=1
  Selector4 : Selector  InputPortWidth=17  IndexOptions=Index vector (dialog)  Indices=[14:17]  OutputSizes=1
  StepAgl/SpeedDownRatio : Gain  Gain=QV_StepAgl./QV_SpdDownRatio
  Subsystem : Subsystem
      mask Display: disp('StTimeStamp')
  Subsystem3 : Subsystem
  Sum : Sum  Inputs=++|
  deg2rad : Gain  Gain=pi/180
  Data_Motor_out : Outport
  SADA_Agl/w/a : Outport  Port=2
  tag scope: Cmd_QV_Proj=global, DataSource_QV_Proj=global, FCAgl_QV_Proj=global, HE1State_QV_Proj=global, HE2State_QV_Proj=global, MotorAgl_QV_Proj=global, Tc_QV_Proj=global
  wires:
  Limit±180deg/1(Out1) -> Sum/1, QV_A_RotUnitQV/1, Subsystem3/1(In1)
  Constant/1 -> Sum/2
  Fre_QV/1(out) -> StepAgl/SpeedDownRatio/1
  Mod/1 -> [MotorAgl_QV_Proj]
  Subsystem3/1(DATA_Motor_HE1Sta) -> [HE1State_QV_Proj]
  Cmd_Motor_in/1 -> [Cmd_QV_Proj]
  Selector1/1 -> SADA_Agl/w/a/1
  AttReset/1 -> Mux2/2
  Constant5/1 -> Mod/2
  Sum/1 -> Mod/1
  "QV_A_RotUnitQV "/1 -> Mux2/3
  Selector4/1 -> [DataSource_QV_Proj], Mux2/4
  "QV_A_DriveRotunit "/1 -> Mux2/5
  QV_A_DriveRotUnit/1 -> Integrator/1
  Integrator/1 -> Limit±180deg/1(In1)
  MATLAB Function4/2(InitialAgl) -> Integrator/3
  Selector2/1 -> "QV_A_RotUnitQV "/1
  Mux2/1 -> MATLAB Function4/1(u)
  Selector/1 -> Mux2/1
  Agl2Agl/w/a/1(Out1) -> Selector1/1
  deg2rad/1 -> Agl2Agl/w/a/1(In1)
  QV_A_RotUnitQV/1 -> deg2rad/1
  MATLAB Function4/1(Tc_level) -> Integrator/2
  TC_Motor_in/1 -> Selector/1, Selector3/1, Selector4/1, Selector2/1
  Subsystem3/2(DATA_Motor_HE2Sta) -> [HE2State_QV_Proj]
  QVAgl_FC/1 -> [FCAgl_QV_Proj], "QV_A_DriveRotunit "/1
  StepAgl/SpeedDownRatio/1 -> QV_A_DriveRotUnit/1
  UTC_1970/1 -> Subsystem/1(UTC_1970)
  Data_QV/1(out) -> Mux/2
  Subsystem/1(St_Time) -> Mux/1
  Mux/1 -> Data_Motor_out/1
  Selector3/1 -> [Tc_QV_Proj]

== system GS_model/Subsystem2/Subsystem/Actuator/Motor/SADA ==
  note: Agl/w/a_A
      | Agl/w/a_B
      | Agl/w/a_C
      | Agl/w/a_D
      | Agl/w/a_E
      | Agl/w/a_F
  note: Agl_A/B/C/D/E/F
      | W_A/B/C/D/E/F
      | a_A/B/C/D/E/F
  TC_Motor_in : Inport
  Cmd_Motor_in : Inport  Port=2
  AttReset : Inport  Port=3
  SADAAgl_FC : Inport  Port=4
  UTC_1970 : Inport  Port=5
  Agl2Agl/w/a : Subsystem
  Constant : Constant  Value=SADA_XbLw_Value
  Constant5 : Constant  Value=360
  Data_SADA : Subsystem
  Fre_SADA : Subsystem
  Integrator : Integrator  ExternalReset=level  InitialConditionSource=external  LimitOutput=on  UpperSaturationLimit=max([(SADA_A_RotUnitSADA.*SADA_PosLocationLimit_Real) (SADA_A_RotUnitSADA.*SADA_NegLocationLimit_Real)],[],2)  LowerSaturationLimit=min([(SADA_A_RotUnitSADA.*SADA_PosLocationLimit_Real) (SADA_A_RotUnitSADA.*SADA_NegLocationLimit_Real)],[],2)
  Limit±180deg : Subsystem
  MATLAB Function4 : MATLAB Function  TreatAsAtomicUnit=on
  Mod : Math  Operator=mod  SaturateOnIntegerOverflow=on
  Mux : Mux  Inputs=2
  Mux2 : Mux  Inputs=5
  SADA_A_DriveRotUnit : Gain  Gain=SADA_A_DriveRotUnit  SaturateOnIntegerOverflow=on  OutDataTypeStr=Inherit: Same as input  ParamDataTypeStr=Inherit: Same as input
  SADA_A_DriveRotunit1 : Gain  Gain=SADA_A_DriveRotUnit  SaturateOnIntegerOverflow=on  OutDataTypeStr=Inherit: Same as input  ParamDataTypeStr=Inherit: Same as input
  SADA_A_RotUnitSADA : Gain  Gain=SADA_A_RotUnitSADA  SaturateOnIntegerOverflow=on  OutDataTypeStr=Inherit: Same as input  ParamDataTypeStr=Inherit: Same as input
  SADA_A_RotUnitSADA1 : Gain  Gain=SADA_A_RotUnitSADA  SaturateOnIntegerOverflow=on  OutDataTypeStr=Inherit: Same as input  ParamDataTypeStr=Inherit: Same as input
  Selector : Selector  InputPortWidth=29  IndexOptions=Index vector (dialog)  Indices=[11:17]  OutputSizes=1
  Selector1 : Selector  InputPortWidth=18  IndexOptions=Index vector (dialog)  Indices=[1 7 13 2 8 14 3 9 15 4 10 16 5 11 17 6 12 18]  OutputSizes=1
  Selector2 : Selector  InputPortWidth=29  IndexOptions=Index vector (dialog)  Indices=[18:23]  OutputSizes=1
  Selector3 : Selector  InputPortWidth=29  IndexOptions=Index vector (dialog)  Indices=[1:17]  OutputSizes=1
  Selector4 : Selector  InputPortWidth=29  IndexOptions=Index vector (dialog)  Indices=[24:29]  OutputSizes=1
  Selector5 : Selector  InputPortWidth=18  IndexOptions=Index vector (dialog)  Indices=1:6  OutputSizes=1
  StepAgl/SpeedDownRatio : Gain  Gain=SADA_StepAgl./SADA_SpdDownRatio
  Subsystem : Subsystem
      mask Display: disp('StTimeStamp')
  Subsystem3 : Subsystem
  Sum : Sum  Inputs=++|
  deg2rad : Gain  Gain=pi/180
  Data_Motor_out : Outport
  SADA_Agl/w/a : Outport  Port=2
  tag scope: Cmd_SADA_Proj=global, DataSource_SADA_Proj=global, FCAgl_SADA_Proj=global, HE1State_SADA_Proj=global, HE2State_SADA_Proj=global, MotorAgl_SADA_Proj=global, TM_SADA_Agl=global, Tc_SADA_Proj=global
  wires:
  SADAAgl_FC/1 -> [FCAgl_SADA_Proj], SADA_A_DriveRotunit1/1  "6"
  StepAgl/SpeedDownRatio/1 -> SADA_A_DriveRotUnit/1
  Subsystem3/2(DATA_Motor_HE2Sta) -> [HE2State_SADA_Proj]
  TC_Motor_in/1 -> Selector4/1, Selector/1, Selector3/1, Selector2/1
  MATLAB Function4/1(Tc_level) -> Integrator/2
  SADA_A_RotUnitSADA/1 -> deg2rad/1
  deg2rad/1 -> Agl2Agl/w/a/1(In1)
  Agl2Agl/w/a/1(Out1) -> Selector5/1, Selector1/1
  Selector/1 -> Mux2/1  "7"
  Mux2/1 -> MATLAB Function4/1(u)
  Selector2/1 -> SADA_A_RotUnitSADA1/1
  MATLAB Function4/2(InitialAgl) -> Integrator/3
  Integrator/1 -> Limit±180deg/1(In1)
  SADA_A_DriveRotUnit/1 -> Integrator/1
  SADA_A_DriveRotunit1/1 -> Mux2/5
  Selector4/1 -> [DataSource_SADA_Proj], Mux2/4  "6"
  SADA_A_RotUnitSADA1/1 -> Mux2/3  "6"
  Sum/1 -> Mod/1
  Constant5/1 -> Mod/2
  AttReset/1 -> Mux2/2  "1"
  Selector1/1 -> SADA_Agl/w/a/1
  Cmd_Motor_in/1 -> [Cmd_SADA_Proj]
  Subsystem3/1(DATA_Motor_HE1Sta) -> [HE1State_SADA_Proj]
  Mod/1 -> [MotorAgl_SADA_Proj]
  Fre_SADA/1(out) -> StepAgl/SpeedDownRatio/1
  Constant/1 -> Sum/2
  Limit±180deg/1(Out1) -> Subsystem3/1(In1), SADA_A_RotUnitSADA/1, Sum/1
  UTC_1970/1 -> Subsystem/1(UTC_1970)
  Subsystem/1(St_Time) -> Mux/1
  Data_SADA/1(out) -> Mux/2
  Mux/1 -> Data_Motor_out/1
  Selector3/1 -> [Tc_SADA_Proj]  "17"
  Selector5/1 -> [TM_SADA_Agl]

== system GS_model/Subsystem2/Subsystem/PhysicsModel/DynModel/AngularMomentumConservation ==
  note: +wXHw?
  Qib : Inport
  Wbi_b : Inport  Port=2
  Ib : Inport  Port=3
  Hw_b : Inport  Port=4
  MatrixMultiply{,1..6} (7 alike) : Product  Multiplication=Matrix(*)
  Quaternions to Direction Cosine Matrix : sharedtransform/Quaternions to  Direction Cosine Matrix  aMode=aMode
      settings: SourceProductBaseCode=AE,PW,MT,VE,VP
  Scope2 : Scope
  Scope3 : Scope
  Sqrt : Sqrt  SaturateOnIntegerOverflow=on
  Square : Math  Operator=square  SaturateOnIntegerOverflow=on
  Sum : Sum  Inputs=|++
  Sum of Elements : Sum  Inputs=+
  Sum2 : Sum  Inputs=|++
  Transpose : Math  Operator=transpose  SaturateOnIntegerOverflow=on
  H_i : Outport
  |H_i| : Outport  Port=2
  wires:
  Qib/1 -> Quaternions to Direction Cosine Matrix/1
  Wbi_b/1 -> MatrixMultiply5/2, MatrixMultiply2/2
  Quaternions to Direction Cosine Matrix/1 -> MatrixMultiply1/2, Transpose/1
  Ib/1 -> MatrixMultiply5/1, MatrixMultiply/2
  MatrixMultiply/1 -> MatrixMultiply1/1
  MatrixMultiply1/1 -> MatrixMultiply3/1
  MatrixMultiply2/1 -> MatrixMultiply3/2
  Hw_b/1 -> Scope2/1, Sum2/2, MatrixMultiply4/2
  Transpose/1 -> MatrixMultiply6/1, MatrixMultiply4/1, MatrixMultiply2/1, MatrixMultiply/1
  MatrixMultiply3/1 -> Sum/1
  MatrixMultiply4/1 -> Sum/2
  MatrixMultiply5/1 -> Sum2/1
  Sum2/1 -> MatrixMultiply6/2
  MatrixMultiply6/1 -> Scope3/1
  Sum/1 -> Square/1, H_i/1
  Sum of Elements/1 -> Sqrt/1
  Square/1 -> Sum of Elements/1
  Sqrt/1 -> |H_i|/1

== system GS_model/Subsystem2/Subsystem/PhysicsModel/DynModel/Att：ECEF2VVLH ==
  Qib : Inport
  wbi_b : Inport  Port=2
  w00 : Inport  Port=3
  Qio : Inport  Port=4
  ECI TO ORBIT : Subsystem
  Quaternion Inverse : aerolibutil/Quaternion Inverse
  Quaternion Multiplication1 : aerolibutil/Quaternion Multiplication
  Quaternions to Direction Cosine Matrix : sharedtransform/Quaternions to  Direction Cosine Matrix  aMode=aMode
      settings: SourceProductBaseCode=AE,PW,MT,VE,VP
  Qob : Outport
  wbo_b : Outport  Port=2
  wires:
  Qio/1 -> Quaternion Inverse/1
  Quaternions to Direction Cosine Matrix/1 -> ECI TO ORBIT/3(Abo)
  w00/1 -> ECI TO ORBIT/2(w00)
  Quaternion Multiplication1/1 -> Quaternions to Direction Cosine Matrix/1, Qob/1
  ECI TO ORBIT/1(wbo(b)) -> wbo_b/1
  wbi_b/1 -> ECI TO ORBIT/1(wbi(b))
  Quaternion Inverse/1 -> Quaternion Multiplication1/1
  Qib/1 -> Quaternion Multiplication1/2

== system GS_model/Subsystem2/Subsystem/PhysicsModel/DynModel/EulerAngle_Inertial ==
  Asc : Inport
  Dec : Inport  Port=2
  Qib : Inport  Port=3
  Constant : Constant  Value=0
  Constant1 : Constant  Value=pi
  Mux : Mux  Inputs=3
  Quaternion Inverse : aerolibutil/Quaternion Inverse
  Quaternion Multiplication : aerolibutil/Quaternion Multiplication
  Quaternions to Rotation Angles : sharedtransform/Quaternions to Rotation Angles  rotationOrder=ZYX  aMode=aMode
      settings: SourceProductBaseCode=AE,PW,MT,VE,VP
  Rotation Angles to Quaternions : sharedtransform/Rotation Angles to Quaternions  rotationOrder=ZYX  aMode=aMode
      settings: SourceProductBaseCode=AE,PW,MT,VE,VP
  Selector1 : Selector  InputPortWidth=3  IndexOptions=Index vector (dialog)  Indices=[3 2 1]  OutputSizes=1
  Sum : Sum  Inputs=++|
  EulerAngle_Inertial : Outport
  wires:
  Rotation Angles to Quaternions/1 -> Quaternion Inverse/1
  Qib/1 -> Quaternion Multiplication/2
  Dec/1 -> Mux/2
  Constant/1 -> Mux/3
  Mux/1 -> Rotation Angles to Quaternions/1
  Quaternion Multiplication/1 -> Quaternions to Rotation Angles/1
  Quaternions to Rotation Angles/1 -> Selector1/1
  Asc/1 -> Sum/2
  Sum/1 -> Mux/1
  Constant1/1 -> Sum/1
  Quaternion Inverse/1 -> Quaternion Multiplication/1
  Selector1/1 -> EulerAngle_Inertial/1

== system GS_model/Subsystem2/Subsystem/PhysicsModel/DynModel/FlexDynModel ==
  Reset_in : Inport
  Hw_in : Inport  Port=2  PortDimensions=3
  dHw_in : Inport  Port=3  PortDimensions=3
  T(b)_in : Inport  Port=4  PortDimensions=3
  Agl_Qio_in : Inport  Port=5
  Att0_in : Inport  Port=6
  RV0_in : Inport  Port=7
  F(i)_in : Inport  Port=8  PortDimensions=3
  SADA_Agl/w/a_a/p_in : Inport  Port=9
  Tc_MassPropertySet_in : Inport  Port=10  PortDimensions=4
  Spread_in : Inport  Port=11  PortDimensions=8
  Agl_Qib : Subsystem
  Cent : Subsystem
  I : Subsystem
  Quaternions to Rotation Angles : sharedtransform/Quaternions to Rotation Angles  rotationOrder=ZYX  aMode=aMode
      settings: SourceProductBaseCode=AE,PW,MT,VE,VP
  R : Subsystem
  V : Subsystem
  dq : Subsystem
  q : Subsystem
  wbi : Subsystem
  R_out : Outport
  V_out : Outport  Port=2
  Agl_Qib_out : Outport  Port=3
  wbi_out : Outport  Port=4
  q_out : Outport  Port=5
  dq_out : Outport  Port=6
  I_out : Outport  Port=7
  Cent_out : Outport  Port=8
  tag scope: Agl_Qio_Proj=global, Att0_Proj=global, F_i_Proj=global, Hw_Proj=global, RV0_Proj=global, Reset_Proj=global, SADA_Aglwa_ap_Proj=global, Spread_Proj=global, T_b_Proj=global, Tc_MassPropertySet_Proj=global, dHw_Proj=global
  wires:
  RV0_in/1 -> [RV0_Proj]
  Att0_in/1 -> [Att0_Proj]
  F(i)_in/1 -> [F_i_Proj]
  T(b)_in/1 -> [T_b_Proj]
  SADA_Agl/w/a_a/p_in/1 -> [SADA_Aglwa_ap_Proj]
  Hw_in/1 -> [Hw_Proj]
  dHw_in/1 -> [dHw_Proj]
  Tc_MassPropertySet_in/1 -> [Tc_MassPropertySet_Proj]
  Agl_Qio_in/1 -> Quaternions to Rotation Angles/1
  V/1(out) -> V_out/1
  wbi/1(out) -> wbi_out/1
  dq/1(out) -> dq_out/1
  q/1(out) -> q_out/1
  Cent/1(out) -> Cent_out/1
  I/1(out) -> I_out/1
  Agl_Qib/1(out) -> Agl_Qib_out/1
  R/1(out) -> R_out/1
  Quaternions to Rotation Angles/1 -> [Agl_Qio_Proj]
  Spread_in/1 -> [Spread_Proj]
  Reset_in/1 -> [Reset_Proj]

== system GS_model/Subsystem2/Subsystem/PhysicsModel/Environment/Air Torque Subsystem ==
  note: Aib
  note: fa=-0.5Cd*rou*vs
  V84_i : Inport
  Abi : Inport  Port=2
  R_Sun : Inport  Port=3
  Abp_PY : Inport  Port=4
  Abp_NY : Inport  Port=5
  Cent : Inport  Port=6
  UnlockSpread : Inport  Port=7
  TC_AirDragCoff : Inport  Port=8
  R_i : Inport  Port=9
  Gain : Gain  Gain=-Cd/2
  Math Function : Math  Operator=transpose  SaturateOnIntegerOverflow=on
  Product : Product  Multiplication=Matrix(*)  SaturateOnIntegerOverflow=on  OutDataTypeStr=Inherit: Same as first input
  Product1 : Product  Multiplication=Matrix(*)  SaturateOnIntegerOverflow=on  OutDataTypeStr=Inherit: Same as first input
  Product2 : Product  Inputs=3  SaturateOnIntegerOverflow=on  OutDataTypeStr=Inherit: Same as first input
  Subsystem : Subsystem
  satalite board : Subsystem
  Fa(i) : Outport
  Ta(b) : Outport  Port=2
  wires:
  Abi/1 -> Product/1, Math Function/1
  V84_i/1 -> Product/2
  Product/1 -> satalite board/1("[Vs]b"), Product2/1
  Product1/1 -> Fa(i)/1
  Product2/1 -> satalite board/2(Fa')
  Abp_PY/1 -> satalite board/3(Abp_PY)
  Math Function/1 -> Product1/1
  satalite board/1(F_a(b)) -> Product1/2
  satalite board/2(T_a(b)) -> Ta(b)/1
  Abp_NY/1 -> satalite board/4(Abp_NY)
  Cent/1 -> satalite board/5(Cent)
  R_Sun/1 -> Subsystem/1(Sun Vector in J2000)
  Gain/1 -> Product2/2
  Subsystem/1(rou) -> Product2/3
  UnlockSpread/1 -> satalite board/6(UnlockSpread)
  TC_AirDragCoff/1 -> Gain/1
  R_i/1 -> Subsystem/2(Earth Vector in J2000)

== system GS_model/Subsystem2/Subsystem/PhysicsModel/Environment/GeoMagTorqueModel ==
  note: Gs
  note: M
  note: B
  Bb : Inport
  M_Mt3 : Inport  Port=2
  Tc_RemainMag : Inport  Port=3
  3x3 Cross Product : sharedutil/3x3 Cross Product  aMode=aMode
      settings: SourceProductBaseCode=AE,PW,MT,VE,VP
  3x3 Cross Product1 : sharedutil/3x3 Cross Product  aMode=aMode
      settings: SourceProductBaseCode=AE,PW,MT,VE,VP
  Gain1 : Gain  Gain=1e-4
  T_RemainMag : Outport  PortDimensions=3
  Tc_Mag : Outport  Port=2  PortDimensions=3
  wires:
  3x3 Cross Product/1 -> T_RemainMag/1
  Bb/1 -> Gain1/1
  Tc_RemainMag/1 -> 3x3 Cross Product/1
  M_Mt3/1 -> 3x3 Cross Product1/1
  Gain1/1 -> 3x3 Cross Product1/2, 3x3 Cross Product/2
  3x3 Cross Product1/1 -> Tc_Mag/1

== system GS_model/Subsystem2/Subsystem/PhysicsModel/Environment/Gravity Torque Subsystem ==
  w0 : Inport
  Abo : Inport  Port=2
  I0 : Inport  Port=3
  3*w0^2 : Gain  Gain=3  SaturateOnIntegerOverflow=on  OutDataTypeStr=Inherit: Same as input  ParamDataTypeStr=Inherit: Same as input
  3x3 Cross Product : sharedutil/3x3 Cross Product  aMode=aMode
      settings: SourceProductBaseCode=AE,PW,MT,VE,VP
  Math Function : Math  Operator=magnitude^2  SaturateOnIntegerOverflow=on
  Product : Product
  Product1 : Product  Multiplication=Matrix(*)  SaturateOnIntegerOverflow=on  InputSameDT=on  OutDataTypeStr=Inherit: Same as first input
  Product3 : Product  Multiplication=Matrix(*)  SaturateOnIntegerOverflow=on  InputSameDT=on  OutDataTypeStr=Inherit: Same as first input
  R0(o) : Constant  Value=[0;0;1]  VectorParams1D=off
  Tgravity : Outport
  wires:
  R0(o)/1 -> Product1/2
  Product3/1 -> 3x3 Cross Product/2
  Product1/1 -> 3x3 Cross Product/1, Product3/2
  I0/1 -> Product3/1
  Abo/1 -> Product1/1
  w0/1 -> Math Function/1
  Math Function/1 -> 3*w0^2/1
  3*w0^2/1 -> Product/1
  3x3 Cross Product/1 -> Product/2
  Product/1 -> Tgravity/1

== system GS_model/Subsystem2/Subsystem/PhysicsModel/Environment/J21 ==
  A_fi : Inport
  R84 : Inport  Port=2  PortDimensions=[3 1]
  Math Function1 : Math  Operator=transpose  SaturateOnIntegerOverflow=on
  Math Function2 : Math  Operator=transpose  SaturateOnIntegerOverflow=on
  Math Function3 : Math  Operator=transpose  SaturateOnIntegerOverflow=on
  Product3 : Product  Multiplication=Matrix(*)
  Spherical Harmonic Gravity Model1 : aerolibgravity2/Spherical Harmonic Gravity Model  units=Metric (MKS)  degree=21  action=Warning  ptype=EGM2008  datafile='aerogmm2b.mat'
      settings: SourceProductBaseCode=AE
  a : Outport
  wires:
  Spherical Harmonic Gravity Model1/1 -> Math Function1/1
  Math Function3/1 -> Product3/1
  A_fi/1 -> Math Function3/1
  Math Function1/1 -> Product3/2
  Product3/1 -> a/1
  R84/1 -> Math Function2/1
  Math Function2/1 -> Spherical Harmonic Gravity Model1/1

== system GS_model/Subsystem2/Subsystem/PhysicsModel/Environment/MagneticCal ==
  note: NED(NorthEastDown)
  note: Longitude
  note: Latitude
  LBH_Geodetic : Inport
  LB_Geocentric : Inport  Port=2
  Orbit : Inport  Port=3
  Abo : Inport  Port=4
  RV_f : Inport  Port=5
  B : Scope  NumInputPorts=2
  Demux : Demux  Outputs=2
  Gain : Gain  Gain=RAD2DEG
  MATLAB Function : MATLAB Function  TreatAsAtomicUnit=on
  Multiply : Product  Commented=on  Multiplication=Matrix(*)
  Multiply1 : Product  Multiplication=Matrix(*)
  Selector : Selector  InputPortWidth=3  IndexOptions=Index vector (dialog)  Indices=[2 1]  OutputSizes=1
  Selector1 : Selector  InputPortWidth=3  IndexOptions=Index vector (dialog)  Indices=3  OutputSizes=1
  Subsystem1 : Subsystem
  World Magnetic Model 2015 : aerolibgravity2/World Magnetic Model 2015  units=Metric (MKS)  time_in=off  month=January  day=1  year=2015  action=Error  h_out=off  dec_out=off  inc_out=off  ti_out=off
      settings: SourceProductBaseCode=AE
  nT2Gs : Gain  Commented=on  Gain=1e-5
  Bb : Outport
  wires:
  Selector1/1 -> World Magnetic Model 2015/1
  LBH_Geodetic/1 -> Selector1/1, Selector/1
  nT2Gs/1 -> Multiply/2
  Gain/1 -> Demux/1
  Selector/1 -> Gain/1
  Abo/1 -> Multiply1/1
  Multiply1/1 -> Bb/1
  Subsystem1/1(Aop) -> Multiply/1
  LB_Geocentric/1 -> MATLAB Function/1(LBH_Geocentric), Subsystem1/1(LB_Geocentric)
  MATLAB Function/1(Mag_VVLH) -> B/2, Multiply1/2
  Demux/1 -> World Magnetic Model 2015/2
  Demux/2 -> World Magnetic Model 2015/3
  World Magnetic Model 2015/1 -> nT2Gs/1
  RV_f/1 -> MATLAB Function/2(fRV)
  Orbit/1 -> Subsystem1/2(Orbit)
  Multiply/1 -> B/1

== system GS_model/Subsystem2/Subsystem/PhysicsModel/Environment/Sun  press torque ==
  Abi : Inport
  R_Sun : Inport  Port=2
  Abp_PY : Inport  Port=3
  Abp_NY : Inport  Port=4
  Cent : Inport  Port=5
  UnlockSpread : Inport  Port=6
  TC_SunPressCoeff : Inport  Port=7
  Sunshine : Inport  Port=8
  MatrixMultiply : Product  Multiplication=Matrix(*)
  MatrixMultiply1 : Product  Multiplication=Matrix(*)
  Normalize Vector : vrlib/Utilities/Normalize Vector  maxzero=0
  Panel Angle : Subsystem
  Sun  press torque2 : Subsystem  TreatAsAtomicUnit=on
  Terminator : Terminator
  Transpose : Math  Operator=transpose  SaturateOnIntegerOverflow=on
  Fs(i) : Outport
  Ts(b) : Outport  Port=2
  wires:
  Sunshine/1 -> Sun  press torque2/5(IfSeeSun)
  Sun  press torque2/2(T_sun) -> Ts(b)/1
  MatrixMultiply1/1 -> Fs(i)/1
  Sun  press torque2/1(F_sun) -> MatrixMultiply1/2
  Abp_PY/1 -> Sun  press torque2/2(Abp_PY)
  Panel Angle/1(PanelAngle) -> Terminator/1
  Cent/1 -> Sun  press torque2/4(Cent)
  UnlockSpread/1 -> Sun  press torque2/1(UnlockSpread)
  Abp_NY/1 -> Sun  press torque2/3(Abp_NY)
  TC_SunPressCoeff/1 -> Sun  press torque2/6(TC_SunPressCoeff)
  R_Sun/1 -> Normalize Vector/1
  MatrixMultiply/1 -> Sun  press torque2/7(Sun(b)), Panel Angle/1(Sun(b))
  Normalize Vector/1 -> MatrixMultiply/2
  Transpose/1 -> MatrixMultiply1/1
  Abi/1 -> MatrixMultiply/1, Transpose/1

== system GS_model/Subsystem2/Subsystem/PhysicsModel/Environment/SunshineAreaCal ==
  R_Sun : Inport
  R_i : Inport  Port=2
  Tc_Sunshine : Inport  Port=3
  1 : Gain
  Demux : Demux  Outputs=2
  Fcn : Fcn  Expr=sqrt(u[1]^2+u[2]^2+u[3]^2)
  Fcn5 : Fcn  Expr=Re/u(1)
  Gain2 : Gain  Gain=-1
  If Action Subsystem2 : Subsystem  TreatAsAtomicUnit=on
  If Action Subsystem5 : Subsystem  TreatAsAtomicUnit=on
  If2 : If  NumInputs=2  IfExpression=u1<=u2
  Math Function1 : Math  Operator=transpose  SaturateOnIntegerOverflow=on
  Merge2 : Merge
  Normalize Vector : vrlib/Utilities/Normalize Vector  maxzero=0
  Normalize Vector1 : vrlib/Utilities/Normalize Vector  maxzero=0
  Product1 : Product  Multiplication=Matrix(*)  SaturateOnIntegerOverflow=on  OutDataTypeStr=Inherit: Same as first input
  Switch : Switch  Criteria=u2 > Threshold  Threshold=0.5
  Trigonometric Function : Trigonometry  Operator=acos
  Trigonometric Function1 : Trigonometry  Operator=asin
  Sunshine : Outport
  wires:
  Trigonometric Function1/1 -> If2/2
  Gain2/1 -> Trigonometric Function/1
  If Action Subsystem2/1(Shadow) -> Merge2/1
  If Action Subsystem5/1(Sunshine) -> Merge2/2
  Normalize Vector1/1 -> Product1/2
  Fcn5/1 -> 1/1
  R_Sun/1 -> Normalize Vector/1
  If2/2 -> If Action Subsystem5/Action
  If2/1 -> If Action Subsystem2/Action
  Trigonometric Function/1 -> If2/1
  1/1 -> Trigonometric Function1/1
  Product1/1 -> Gain2/1
  Math Function1/1 -> Product1/1
  Fcn/1 -> Fcn5/1
  R_i/1 -> Normalize Vector1/1, Fcn/1
  Normalize Vector/1 -> Math Function1/1
  Tc_Sunshine/1 -> Demux/1
  Demux/1 -> Switch/2
  Demux/2 -> Switch/1
  Merge2/1 -> Switch/3
  Switch/1 -> Sunshine/1
